simulink library "INT_APP_PlausBrk"  (R2016b)
settings: Solver=VariableStepAuto  StartTime=0.0  StopTime=10.0  RelTol=1e-3
settings Model: Creator=Administrator  LastModifiedBy=Administrator

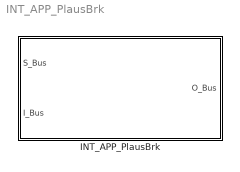
== system INT_APP_PlausBrk ==
  INT_APP_PlausBrk : Subsystem

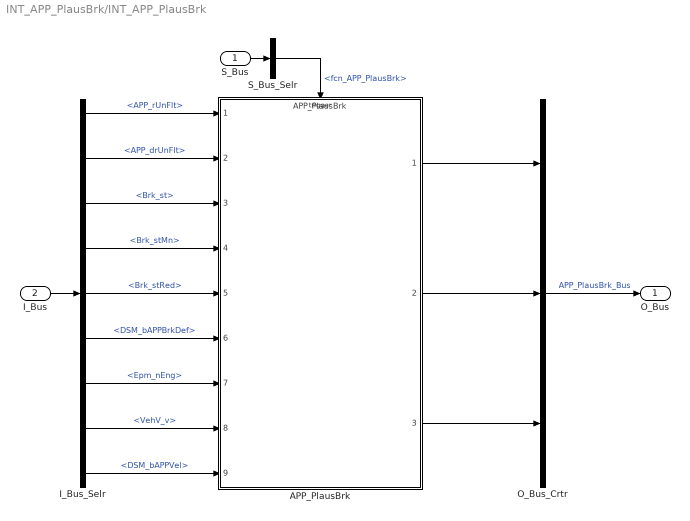
== system INT_APP_PlausBrk/INT_APP_PlausBrk ==
  S_Bus : Inport
  I_Bus : Inport  Port=2
  APP_PlausBrk : ModelReference  ModelNameDialog=APP_PlausBrk  SimulationMode=Normal  ModelReferenceVersion=1.27  TriggerPortName=function  TriggerPortTriggerType=function-call  TriggerPortStatesWhenEnabling=held
  I_Bus_Selr : BusSelector  OutputSignals=APP_rUnFlt,APP_drUnFlt,Brk_st,Brk_stMn,Brk_stRed,DSM_bAPPBrkDef,Epm_nEng,VehV_v,DSM_bAPPVel
  O_Bus_Crtr : BusCreator  Inputs=3
  S_Bus_Selr : BusSelector  OutputSignals=fcn_APP_PlausBrk
  O_Bus : Outport
  wires:
  S_Bus_Selr/1 -> APP_PlausBrk/Trigger  "<fcn_APP_PlausBrk>"
  S_Bus/1 -> S_Bus_Selr/1
  I_Bus/1 -> I_Bus_Selr/1
  I_Bus_Selr/1 -> APP_PlausBrk/1  "<APP_rUnFlt>"
  I_Bus_Selr/2 -> APP_PlausBrk/2  "<APP_drUnFlt>"
  I_Bus_Selr/3 -> APP_PlausBrk/3  "<Brk_st>"
  I_Bus_Selr/4 -> APP_PlausBrk/4  "<Brk_stMn>"
  I_Bus_Selr/5 -> APP_PlausBrk/5  "<Brk_stRed>"
  I_Bus_Selr/6 -> APP_PlausBrk/6  "<DSM_bAPPBrkDef>"
  I_Bus_Selr/7 -> APP_PlausBrk/7  "<Epm_nEng>"
  I_Bus_Selr/8 -> APP_PlausBrk/8  "<VehV_v>"
  I_Bus_Selr/9 -> APP_PlausBrk/9  "<DSM_bAPPVel>"
  O_Bus_Crtr/1 -> O_Bus/1  "APP_PlausBrk_Bus"
  APP_PlausBrk/1 -> O_Bus_Crtr/1
  APP_PlausBrk/2 -> O_Bus_Crtr/2
  APP_PlausBrk/3 -> O_Bus_Crtr/3
